simulink model "CryoDet6"  (R2015a)
settings: Solver=ode45  SolverMode=SingleTasking  StartTime=0.0  StopTime=1e-3  MaxStep=Tclk/8  RelTol=1e-3
values from neighbouring files (symbols this model uses):
  Fclk = Fadc/2    (= 185000000)    [setupCryoFPGA.m]    (also in setupCryoNew.m)
  noise = exp(1i*phi)    [setupCryoFPGA.m]    (also in setupCryoNew.m = exp(2i*pi*rand(1, noiseLen)))
  noiseLen = 128    [setupCryoFPGA.m]    (also in setupCryoNew.m)
  noiseSteps = 32    [setupCryoFPGA.m]    (also in setupCryoNew.m)
  notch = tf( [1 a*wNotch/Q wNotch^2], [1 wNotch/Q wNotch^2])    [setupCryoFPGA.m]    (also in setupCryoNew.m)
  notch2 = tf( [1 a*wNotch/Q wNotch^2], [1 wNotch/Q wNotch^2])    [setupCryoFPGA.m]    (also in setupCryoNew.m)
  setupVers = 5    [setupCryoFPGA.m]    (also in setupCryoNew.m = 21)
  Tclk = 1/Fclk    (= 5.40540540541e-09)    [setupCryoFPGA.m]    (also in setupCryoNew.m)
  wTs1 = w1*Ts1    (= 0.0271705310581)    [setupCryoFPGA.m]
undefined symbols (not defined in the file or in its folder): AXI4, Lite, xlipgetpartsetting
libraries: xbsIndex_r4 x516, simulink x1
(part 3 of 6)

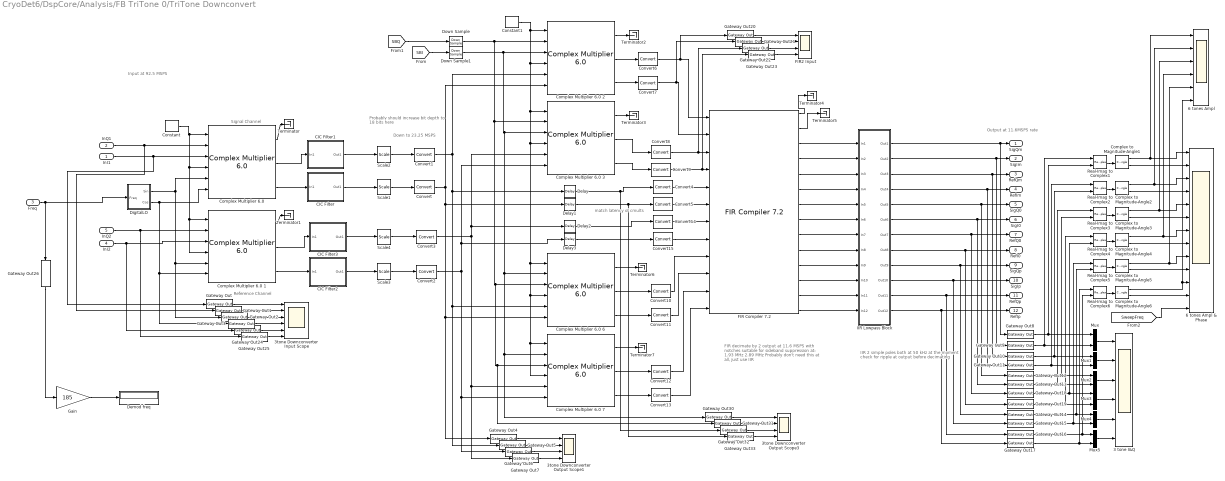
== system CryoDet6/DspCore/Analysis/FB TriTone 0/TriTone Downconvert ==
  note: Probably should increase bit depth
      | to 18 bits here
  note: IIR 2 simple poles
      | both at 50 kHz at the moment
      | check for ripple at output before decimating
  note: FIR decimate by 2
      | output at 11.6 MSPS
      | with notches suitable for
      | sideband suppression at:
      | 1.93 MHz
      | 2.89 MHz
      |
      | Probably don't need this at all, just use IIR
  note: Output at 11.6MSPS rate
  note: Down to 23.25 MSPS
  note: Input at 92.5 MSPS
  note: Reference Channel
  note: Signal Channel
  note: match latency
      | of cmults
  InI1 : Inport
  InQ1 : Inport  Port=2
  Freq : Inport  Port=3
  InI2 : Inport  Port=4
  InQ2 : Inport  Port=5
  3 tone I&Q : Scope  NumInputPorts=6
      settings: TimeRange=0.0002910432432432433  YMin=-0.008~-0.003~-0.15~-0.025~-0.0075~-0.0075  YMax=0.005~0.004~0.15~0.225~0.0075~0.01  SaveName=ScopeData7  MaxDataPoints=10000  SampleInput=on  SampleTime=Tclk
  3tone Downconverter Input Scope : Scope  NumInputPorts=6
      settings: TimeRange=1e-05  YMin=-0.75~-0.75~-1~-1~-0.5~-0.5  YMax=0.75~0.75~1~1~0.4~0.5  SaveName=ScopeData4
  3tone Downconverter Output Scope1 : Scope  NumInputPorts=4
      settings: TimeRange=0.000216172972972973  YMin=0.05~-0.2~-0.7000000000000001~-0.2  YMax=0.25~0.2~-0.2000000000000001~0.6000000000000001  SaveName=ScopeData6
  3tone Downconverter Output Scope3 : Scope  NumInputPorts=4
      settings: TimeRange=9.98918918918919e-06  YMin=-1~-1~-1~-1  YMax=1~1~1~1  SaveName=ScopeData13
  6 tones Ampl : Scope  NumInputPorts=6
      settings: TimeRange=0.0001119135135135135  YMin=0.00025~0.00026~0.182~0.279182~0.0002~0.00026  YMax=0.00175~0.00039~0.187~0.279184~0.0014~0.00039  SaveName=TonePandA1  DataFormat=Structure  MaxDataPoints=10000  SampleInput=on  SampleTime=Tclk*64
  6 tones Ampl & Phase : Scope  NumInputPorts=13
      settings: TimeRange=0.0001119135135135135  YMin=0.048259~0.825~0.0490775~-1.275~0.100188~0.5~0.502076~-3~0.05489~-0.5~0.0557525~-3.125~6.9966e+07  YMax=0.0482615~1~0.0490875~-1.125~0.100192~0.675~0.502082~-2.825~0.0549025~-0.325~0.0557625~-2.975~6.997e+07  SaveName=TonePandA  DataFormat=Structure  MaxDataPoints=10000  SampleInput=on  SampleTime=Tclk*16
  CIC Filter : Subsystem  mask(CIC Filter){input_bitwidth=20, input_binpt=16, filter_type=Decimator, rate_change=4, stages=3, m=1, pipeline=on}
      mask prompts: input_bitwidth "Input Bit Width"; input_binpt "Input Binary Point"; filter_type "Filter Type"; rate_change "Sample Rate Change"; stages "Number of Stages"; m "Differential Delay"; pipeline "Pipeline Differentiators"
      mask help: Cascaded Integrated Comb (CIC) Filter
      mask init:
      | % CIC Single Channel v1.0
      | % Set Block Logo
      | sav_gcb=gcb;
      | [bg,fg] = xlcmap('XBlock',0);
      | iPos = get_param(sav_gcb,'Position');
      | iWidth=iPos(3)-iPos(1); iHeight=iPos(4)-iPos(2);
      | iCx=iWidth/2;
      | iCy=iHeight/2;
      | [logoX, logoY] = xlogo(iPos);
      | 
      | % Determine previous filter type and number of stages
      | prev_stages_list = find_system(sav_gcb, 'lookUnderMasks', 'all', 'FollowLinks', 'on', 'Regexp', 'on', 'Name', '^Integrator*'); %this is a cell array
      | prev_stages = length(prev_stages_list);
      | 
      | prev_filter_list = find_system(sav_gcb, 'lookUnderMasks', 'all', 'FollowLinks', 'on', 'Regexp', 'on', 'Name', '^Up Sample*'); %this is a cell array
      | if (isempty(prev_filter_list))
      |     prev_filter_list = find_system(sav_gcb, 'lookUnderMasks', 'all', 'FollowLinks', 'on', 'Regexp', 'on', 'Name', '^Down Sample*'); %this is a cell array
      |     if (isempty(prev_filter_list))
      |         errordlg('Previous Filter Type could not be determined')
      |     else
      |         prev_filter_type = 2;
      |     end
      | else
      |     prev_filter_type = 1;
      | end
      |   
      |   
      | % Print label on the block
      | if(filter_type == 2)
      |    cic_str = sprintf('%d-Stage\n CIC\n%d:1 Decimator',stages, rate_change);
      | else
      |    cic_str = sprintf('%d-Stage\n CIC\n1:%d Interpolator',stages, rate_change);	
      | end
      | 
      | % Make sure the entered values for stages and channels are positive integers
      | nstages = round(sum(abs(stages)));
      | 
      | % issue an error if the number of stages entered is zero
      | if (nstages == 0)
      | 	nstages = prev_stages;
      | 	errordlg('Number of Stages must be more than zero')
      | end
      | 
      | if (nstages == prev_stages) & (filter_type == prev_filter_type)
      |     return
      | end
      | 
      | if(filter_type == 2) % Decimator
      |    if (prev_filter_type == 1) % was interpolator so turn to decimator
      |        for i= 2:prev_stages,
      | 	      delete_line(sav_gcb, ['Integrator' int2str(i-1) '/' int2str(1)], ['Integrator' int2str(i) '/' int2str(1)]);
      | 	      delete_line(sav_gcb, ['Differentiator' int2str(i-1) '/' int2str(1)], ['Differentiator' int2str(i) '/' int2str(1)]);
      |        end
      | 
      |        % disconnect the last blocks in the two sections
      |        delete_line(sav_gcb, ['Differentiator' int2str(prev_stages) '/' int2str(1)], ['Up Sample/1']);
      |        delete_line(sav_gcb, ['Integrator' int2str(prev_stages) '/' int2str(1)], 'Out1/1');
      | 	
      | 	   % delete the line from the Up sampler to the Integrator
      | 	   delete_line(sav_gcb, 'Up Sample/1', 'Integrator1/1'); 
      | 	   delete_line(sav_gcb, 'In1/1', 'Differentiator1/1'); 
      | 	   
      | 	   % Delete the Up Sampler and then replace with an Down Sampler
      | 	   pup = get_param([sav_gcb '/Up Sample'], 'position');
      | 	   delete_block([sav_gcb '/Up Sample']);
      | 	   load_system('xbsIndex_r4');
      | 	   add_block('xbsIndex_r4/Down Sample', [sav_gcb '/Down Sample'], 'sample_ratio', 'rate_change','sample_phase', 'First Value of Frame', 'position', [pup(1), pup(2), pup(3),pup(4)]);
      | 	   
      | 	   % Switch the Integrators and Decimators around
      | 	   for i=1:prev_stages,
      | 		   tempi = get_param([sav_gcb '/Integrator' int2str(i)], 'position');
      | 	       tempd = get_param([sav_gcb '/Differentiator' int2str(i)], 'position');
      | 		   set_param([sav_gcb '/Differentiator' int2str(i)], 'position', [tempi(1), tempi(2), tempi(3), tempi(4)], 'output_bitwidth', 'ceil(stages*log2(rate_change*m) + input_bitwidth)');
      | 		   set_param([sav_gcb '/Integrator' int2str(i)], 'position', [tempd(1), tempd(2), tempd(3), tempd(4)]);
      | 	   end
      | 	   	   	
      | 	   % add back in the lines
      |        add_line(sav_gcb, 'In1/1', 'Integrator1/1', 'autorouting', 'on');
      | 	   add_line(sav_gcb, ['Integrator' int2str(prev_stages) '/1'], 'Down Sample/1', 'autorouting', 'on');
      | 	   add_line(sav_gcb, 'Down Sample/1', 'Differentiator1/1', 'autorouting', 'on');
      | 	   add_line(sav_gcb, ['Differentiator' int2str(prev_stages) '/1'], 'Out1/1', 'autorouting', 'on');
      | 	   for i= 2:prev_stages,
      |           add_line(sav_gcb, ['Integrator' int2str(i-1) '/1'], ['Integrator' int2str(i) '/' int2str(1)], 'autorouting', 'on');
      |           add_line(sav_gcb, ['Differentiator' int2str(i-1) '/1'], ['Differentiator' int2str(i) '/' int2str(1)], 'autorouting', 'on');
      | 	   end
      | 		
      |        %Set the Output bit widths of Differentiator and Integrator stages
      |        set_param([sav_gcb '/Differentiator1'], 'output_bitwidth', 'ceil(stages*log2(rate_change*m) + input_bitwidth)');
      | 	   	   %Set the Output bit width of Integrator stages
      | 	   %Calculate the Interpolator Integrator Output Bit Growth
      |        for i= 1:prev_stages,
      | 			 j = nstages+i;
      | 	         set_param([sav_gcb '/Integrator' int2str(i)], 'output_bitwidth', 'ceil(stages*log2(rate_change*m) + input_bitwidth)');
      |              set_param([sav_gcb '/Differentiator' int2str(i)], 'output_bitwidth', 'ceil(stages*log2(rate_change*m) + input_bitwidth)');
      | 	   end
      | 	   
      |    end
      |    
      |    if (nstages ~= prev_stages)
      |     
      |        % disconnect all the wires from all the blocks
      |        for i= 2:prev_stages,
      | 	      delete_line(sav_gcb, ['Integrator' int2str(i-1) '/' int2str(1)], ['Integrator' int2str(i) '/' int2str(1)]);
      | 	      delete_line(sav_gcb, ['Differentiator' int2str(i-1) '/' int2str(1)], ['Differentiator' int2str(i) '/' int2str(1)]);
      |        end
      | 
      |        % disconnect the last blocks in the two sections
      |        delete_line(sav_gcb, ['Integrator' int2str(prev_stages) '/' int2str(1)], ['Down Sample/1']);
      |        delete_line(sav_gcb, ['Differentiator' int2str(prev_stages) '/' int2str(1)], 'Out1/1');
      | 	
      | 	   % delete the line from the down sampler to the differentiator
      | 	   delete_line(sav_gcb, 'Down Sample/1', 'Differentiator1/1');
      | 	
      | 	   % Remove all the blocks except the first one (as we always will have one)
      |        for i=2:prev_stages,
      | 		  delete_block([sav_gcb '/Differentiator' int2str(i)]);
      | 	      delete_block([sav_gcb '/Integrator' int2str(i)]);
      |        end
      | 	   
      | 	   %Set the Output bit width of Differentiator stages
      |        set_param([sav_gcb '/Differentiator1'], 'output_bitwidth', 'ceil(stages*log2(rate_change*m) + input_bitwidth)');
      | 	   
      | 	   % collect data on the position of existing blocks
      | 	   pi = get_param([sav_gcb '/Integrator1'], 'position');
      | 	   pd = get_param([sav_gcb '/Differentiator1'], 'position');
      | 	   set_param([sav_gcb '/Differentiator1'], 'position', [pi(1)+(nstages+1)*80, pd(2), pi(3)+(nstages+1)*80, pd(4)]);
      | 	   pd = get_param([sav_gcb '/Differentiator1'], 'position');
      | 	
      | 	   % move the current blocks to accomadate for new blocks to be added 
      | 	   pds = get_param([sav_gcb '/Down Sample'], 'position');
      | 	   set_param([sav_gcb '/Down Sample'], 'position', [pi(1)+(nstages)*80, pds(2), pi(3)+(nstages)*80, pds(4)]);
      | 	   
      | 	   po = get_param([sav_gcb '/Out1'], 'position');
      | 	   set_param([sav_gcb '/Out1'], 'position', [pd(1)+(nstages+1)*80, po(2), pd(1)+(po(3)-po(1))+(nstages+1)*80, po(4)]);	
      | 	
      | 	   % add back in the line between the Down Sampler and the 1st Differentiator
      |        add_line(sav_gcb, 'Down Sample/1', ['Differentiator1/' int2str(1)], 'autorouting', 'on');
      | 
      | 	   % Only add blocks if more than one stage is required
      | 	   if (nstages ~= 1)
      | 		
      | 	       % Add in a copy of the first block to make up the required number of stages
      |            for i=2:nstages,
      |                add_block([sav_gcb '/Integrator1'], [sav_gcb '/Integrator' int2str(i)], 'position', [pi(1)+(i-1)*80, pi(2), pi(3)+(i-1)*80, pi(4)]);
      | 		       add_block([sav_gcb '/Differentiator1'], [sav_gcb '/Differentiator' int2str(i)], 'position', [pd(1)+(i-1)*80, pd(2), pd(3)+(i-1)*80, pd(4)]);
      | 	       end
      | 		
      | 	       % Connect up the wires to each block use autorouting
      |            for i= 2:nstages,
      |  		       add_line(sav_gcb, ['Integrator' int2str(i-1) '/' int2str(1)], ['Integrator' int2str(i) '/' int2str(1)], 'autorouting', 'on');
      | 	           add_line(sav_gcb, ['Differentiator' int2str(i-1) '/' int2str(1)], ['Differentiator' int2str(i) '/' int2str(1)], 'autorouting', 'on');
      |            end
      | 	    end
      | 	       % Connect the last blocks in the two sections
      |            add_line(sav_gcb, ['Integrator' int2str(nstages) '/' int2str(1)], ['Down Sample/1'], 'autorouting', 'on');
      |            add_line(sav_gcb, ['Differentiator' int2str(nstages) '/' int2str(1)], ['Out1/1'], 'autorouting', 'on');
      |    end
      | 
      | else % Interpolator
      |    
      | 	
      | 	if (prev_filter_type == 2) % was decimator so turn to interpolator
      | 	
      | 	  % disconnect all the wires from all the blocks
      |        for i= 2:prev_stages,
      | 	      delete_line(sav_gcb, ['Integrator' int2str(i-1) '/' int2str(1)], ['Integrator' int2str(i) '/' int2str(1)]);
      | 	      delete_line(sav_gcb, ['Differentiator' int2str(i-1) '/' int2str(1)], ['Differentiator' int2str(i) '/' int2str(1)]);
      |        end
      | 
      |        % disconnect the last blocks in the two sections
      |        delete_line(sav_gcb, ['Integrator' int2str(prev_stages) '/' int2str(1)], ['Down Sample/1']);
      |        delete_line(sav_gcb, ['Differentiator' int2str(prev_stages) '/' int2str(1)], 'Out1/1');
      | 	
      | 	   % delete the line from the down sampler to the Differentiator
      | 	   delete_line(sav_gcb, 'Down Sample/1', 'Differentiator1/1'); 
      | 	   delete_line(sav_gcb, 'In1/1', 'Integrator1/1'); 
      | 	   
      | 	   % Delete the Down Sampler and then replace with a Up Sampler
      | 	   pdwn = get_param([sav_gcb '/Down Sample'], 'position');
      | 	   delete_block([sav_gcb '/Down Sample']);
      | 	   load_system('xbsIndex_r4');
      | 	   add_block('xbsIndex_r4/Up Sample', [sav_gcb '/Up Sample'], 'sample_ratio', 'rate_change', 'position', [pdwn(1), pdwn(2), pdwn(3), pdwn(4)]);
      | 	   
      | 	   % Switch the Integrators and Decimators around
      | 	   for i=1:prev_stages,
      | 		   tempi = get_param([sav_gcb '/Integrator' int2str(i)], 'position');
      | 	       tempd = get_param([sav_gcb '/Differentiator' int2str(i)], 'position');
      | 		   set_param([sav_gcb '/Differentiator' int2str(i)], 'position', [tempi(1), tempi(2), tempi(3), tempi(4)], 'output_bitwidth', [int2str(i) '+ input_bitwidth']);
      | 		   set_param([sav_gcb '/Integrator' int2str(i)], 'position', [tempd(1), tempd(2), tempd(3), tempd(4)]);
      | 	   end
      | 	   	   	
      | 	   % add back in the lines
      |        add_line(sav_gcb, 'In1/1', 'Differentiator1/1', 'autorouting', 'on');
      | 	   add_line(sav_gcb, ['Differentiator' int2str(prev_stages) '/1'], 'Up Sample/1', 'autorouting', 'on');
      | 	   add_line(sav_gcb, 'Up Sample/1', 'Integrator1/1', 'autorouting', 'on');
      | 	   add_line(sav_gcb, ['Integrator' int2str(prev_stages) '/1'], 'Out1/1', 'autorouting', 'on');
      | 	   for i= 2:prev_stages,
      |           add_line(sav_gcb, ['Integrator' int2str(i-1) '/1'], ['Integrator' int2str(i) '/1'], 'autorouting', 'on');
      |           add_line(sav_gcb, ['Differentiator' int2str(i-1) '/1'], ['Differentiator' int2str(i) '/1'], 'autorouting', 'on');
      | 	   end
      | 	   
      | 	   %Set the Output bit width of Integrator stages
      | 	   %Calculate the Interpolator Integrator Output Bit Growth
      |        for i= 1:prev_stages,
      | 			 j = nstages+i;
      | 	         set_param([sav_gcb '/Integrator' int2str(i)], 'output_bitwidth', ['ceil(log2(2^(2*stages-' int2str(j) ')*(rate_change*m)^(' int2str(j) '-stages)) + input_bitwidth)']);
      | 	   end
      | 		
      |    end
      |    
      | 	
      | 	if (nstages ~= prev_stages)
      |     
      |        % disconnect all the wires from all the blocks
      |        for i= 2:prev_stages,
      | 	      delete_line(sav_gcb, ['Integrator' int2str(i-1) '/' int2str(1)], ['Integrator' int2str(i) '/' int2str(1)]);
      | 	      delete_line(sav_gcb, ['Differentiator' int2str(i-1) '/' int2str(1)], ['Differentiator' int2str(i) '/' int2str(1)]);
      |        end
      | 
      |        % disconnect the last blocks in the two sections
      |        delete_line(sav_gcb, ['Differentiator' int2str(prev_stages) '/' int2str(1)], ['Up Sample/1']);
      |        delete_line(sav_gcb, ['Integrator' int2str(prev_stages) '/' int2str(1)], 'Out1/1');
      |        
      | 	
      | 	   % delete the line from the Up sampler to the Integrator1 for movement later
      | 	   delete_line(sav_gcb, 'Up Sample/1', 'Integrator1/1'); 
      | 	
      | 	   % Remove all the blocks except the first one (as we always will have one)
      |        for i=2:prev_stages,
      | 		  delete_block([sav_gcb '/Differentiator' int2str(i)]);
      | 	      delete_block([sav_gcb '/Integrator' int2str(i)]);
      |        end
      | 	
      | 	   %Set the Output bit width of first Differentiator stage (other are set as copies of this block)
      |        set_param([sav_gcb '/Differentiator1'], 'output_bitwidth', '1 + input_bitwidth');
      | 	   
      | 	   % collect data on the position of existing blocks
      | 	   pi = get_param([sav_gcb '/Integrator1'], 'position');
      | 	   pd = get_param([sav_gcb '/Differentiator1'], 'position');
      | 	   set_param([sav_gcb '/Integrator1'], 'position', [pd(1)+(nstages+1)*80, pi(2), pd(3)+(nstages+1)*80, pi(4)]);
      | 	   pi = get_param([sav_gcb '/Integrator1'], 'position');
      | 	
      | 	   % move the current blocks to accomadate for new blocks to be added 
      | 	   pus = get_param([sav_gcb '/Up Sample'], 'position');
      | 	   set_param([sav_gcb '/Up Sample'], 'position', [pd(1)+(nstages)*80, pus(2), pd(3)+(nstages)*80, pus(4)]);
      | 	
      | 	   po = get_param([sav_gcb '/Out1'], 'position');
      |        set_param([sav_gcb '/Out1'], 'position', [pi(1)+(nstages+1)*80, po(2), pi(1)+(po(3)-po(1))+(nstages+1)*80, po(4)]);	
      |       
      | 	
      | 	   % add back in the line between the Up Sampler and the 1st Integrator1
      | 	   add_line(sav_gcb, 'Up Sample/1', 'Integrator1/1', 'autorouting', 'on');
      | 	   
      | 	   % Only add blocks if more than one stage is required
      | 	   if (nstages ~= 1)
      | 		
      | 	       % Add in a copy of the first block to make up the required number of stages
      |            for i=2:nstages,
      |                add_block([sav_gcb '/Integrator1'], [sav_gcb '/Integrator' int2str(i)], 'position', [pi(1)+(i-1)*80, pi(2), pi(3)+(i-1)*80, pi(4)]);
      | 		       add_block([sav_gcb '/Differentiator1'], [sav_gcb '/Differentiator' int2str(i)], 'position', [pd(1)+(i-1)*80, pd(2), pd(3)+(i-1)*80, pd(4)], 'output_bitwidth', [int2str(i) '+ input_bitwidth']);
      | 	       end
      | 		
      | 	       % Connect up the wires to each block use autorouting
      |            for i= 2:nstages,
      |  		       add_line(sav_gcb, ['Integrator' int2str(i-1) '/' int2str(1)], ['Integrator' int2str(i) '/' int2str(1)], 'autorouting', 'on');
      | 	           add_line(sav_gcb, ['Differentiator' int2str(i-1) '/' int2str(1)], ['Differentiator' int2str(i) '/' int2str(1)], 'autorouting', 'on');
      |            end
      | 	    end
      | 	       % Connect the last blocks in the two sections
      |            add_line(sav_gcb, ['Differentiator' int2str(nstages) '/1'], ['Up Sample/1'], 'autorouting', 'on');
      |            add_line(sav_gcb, ['Integrator' int2str(nstages) '/1'], ['Out1/1'], 'autorouting', 'on');
      | 		   
      | 	     %Set the Output bit width of Integrator stages
      | 	     %Calculate the Interpolator Integrator Output Bit Growth
      |           for i= 1:nstages,
      | 			 j = nstages+i;
      | 	         set_param([sav_gcb '/Integrator' int2str(i)], 'output_bitwidth', ['ceil(log2(2^(2*stages-' int2str(j) ')*(rate_change*m)^(' int2str(j) '-stages)) + input_bitwidth)']);
      | 	      end
      |    end
      | 	  
      | end
      | 
      | 
      | % Set the pipelining to ON or OFF on the differentiators
      | if (pipeline == 0)
      | 	for i= 1:nstages
      | 		set_param([sav_gcb '/Differentiator' int2str(i), '/AddSub'], 'latency', '0')
      | 	end
      | else
      | 	for i= 1:nstages
      | 		set_param([sav_gcb '/Differentiator' int2str(i), '/AddSub'], 'latency' ,'1')
      | 	end
      | end
      settings: CopyFcn=set_param(gcb, 'MaskSelfModifiable', 'on', 'LinkStatus', 'none');
      mask Help: eval('');xlDoc('-book','sysgen','-topic','CIC_Filter');
      mask TypeOptions filter_type: Interpolator | Decimator
      mask TypeOptions m: 1 | 2 | 3 | 4
      mask Display:
      | patch([0 iWidth iWidth 0],[0 0 iHeight iHeight] , bg);
      | patch(logoX,logoY , fg);
      | plot([0 0 iWidth iWidth 0], [0 iHeight iHeight 0 0]);
      | disp(cic_str)
  CIC Filter1 : Subsystem  mask(CIC Filter){input_bitwidth=20, input_binpt=16, filter_type=Decimator, rate_change=4, stages=3, m=1, pipeline=on}
      mask prompts: input_bitwidth "Input Bit Width"; input_binpt "Input Binary Point"; filter_type "Filter Type"; rate_change "Sample Rate Change"; stages "Number of Stages"; m "Differential Delay"; pipeline "Pipeline Differentiators"
      mask help: Cascaded Integrated Comb (CIC) Filter
      mask init: same as CryoDet6/DspCore/Analysis/FB TriTone 0/TriTone Downconvert/CIC Filter
      settings: CopyFcn=set_param(gcb, 'MaskSelfModifiable', 'on', 'LinkStatus', 'none');
      mask Help: eval('');xlDoc('-book','sysgen','-topic','CIC_Filter');
      mask TypeOptions filter_type: Interpolator | Decimator
      mask TypeOptions m: 1 | 2 | 3 | 4
      mask Display:
      | patch([0 iWidth iWidth 0],[0 0 iHeight iHeight] , bg);
      | patch(logoX,logoY , fg);
      | plot([0 0 iWidth iWidth 0], [0 iHeight iHeight 0 0]);
      | disp(cic_str)
  CIC Filter2 : Subsystem  mask(CIC Filter){input_bitwidth=20, input_binpt=16, filter_type=Decimator, rate_change=4, stages=3, m=1, pipeline=on}
      mask prompts: input_bitwidth "Input Bit Width"; input_binpt "Input Binary Point"; filter_type "Filter Type"; rate_change "Sample Rate Change"; stages "Number of Stages"; m "Differential Delay"; pipeline "Pipeline Differentiators"
      mask help: Cascaded Integrated Comb (CIC) Filter
      mask init: same as CryoDet6/DspCore/Analysis/FB TriTone 0/TriTone Downconvert/CIC Filter
      settings: CopyFcn=set_param(gcb, 'MaskSelfModifiable', 'on', 'LinkStatus', 'none');
      mask Help: eval('');xlDoc('-book','sysgen','-topic','CIC_Filter');
      mask TypeOptions filter_type: Interpolator | Decimator
      mask TypeOptions m: 1 | 2 | 3 | 4
      mask Display:
      | patch([0 iWidth iWidth 0],[0 0 iHeight iHeight] , bg);
      | patch(logoX,logoY , fg);
      | plot([0 0 iWidth iWidth 0], [0 iHeight iHeight 0 0]);
      | disp(cic_str)
  CIC Filter3 : Subsystem  mask(CIC Filter){input_bitwidth=20, input_binpt=16, filter_type=Decimator, rate_change=4, stages=3, m=1, pipeline=on}
      mask prompts: input_bitwidth "Input Bit Width"; input_binpt "Input Binary Point"; filter_type "Filter Type"; rate_change "Sample Rate Change"; stages "Number of Stages"; m "Differential Delay"; pipeline "Pipeline Differentiators"
      mask help: Cascaded Integrated Comb (CIC) Filter
      mask init: same as CryoDet6/DspCore/Analysis/FB TriTone 0/TriTone Downconvert/CIC Filter
      settings: CopyFcn=set_param(gcb, 'MaskSelfModifiable', 'on', 'LinkStatus', 'none');
      mask Help: eval('');xlDoc('-book','sysgen','-topic','CIC_Filter');
      mask TypeOptions filter_type: Interpolator | Decimator
      mask TypeOptions m: 1 | 2 | 3 | 4
      mask Display:
      | patch([0 iWidth iWidth 0],[0 0 iHeight iHeight] , bg);
      | patch(logoX,logoY , fg);
      | plot([0 0 iWidth iWidth 0], [0 iHeight iHeight 0 0]);
      | disp(cic_str)
  "Complex Multiplier 6.0 " : xbsIndex_r4/Complex Multiplier 6.0   hasatlast=off  hasatuser=off  atuserwidth=1  hasbtlast=off  hasbtuser=off  btuserwidth=1  multtype=Use_Mults  optimizegoal=Resources  flowcontrol=NonBlocking  outputwidth=20  roundmode=Truncate  hasctrltlast=off  hasctrltuser=off  ctrltuserwidth=1  outtlastbehv=Null  latencyconfig=Automatic  minimumlatency=37  aclken=off  aresetn=off  trim_axipin_name=on  simulation_type=hybrid_sim  simulation_model=sysgen:cmpy_v6_0  data_path_portlist={ 's_axis_a_tdata_real', 's_axis_a_tdata_imag', 's_axis_b_tdata_real', 's_axis_b_tdata_imag', 's_axis_ctrl_tdata_rounding_bit', 'm_axis_dout_tdata_real', 'm_axis_dout_tdata_imag' }  aportwidth=63  bportwidth=63  ip_name=Complex Multiplier  ip_version=6.0  dsptool_ready=true  ipcore_usecache=true  ipcore_useipmodelcache=true  ipcore_verbose=false  ipcore_latency_parameter='minimumlatency'  wrapper_available=true  port_translation_map={ 'aclken' => 'en', 'aresetn' => 'rst'}  block_type=cmpy_v6_0
  Complex Multiplier 6.0 1 : xbsIndex_r4/Complex Multiplier 6.0   hasatlast=off  hasatuser=off  atuserwidth=1  hasbtlast=off  hasbtuser=off  btuserwidth=1  multtype=Use_Mults  optimizegoal=Resources  flowcontrol=NonBlocking  outputwidth=20  roundmode=Truncate  hasctrltlast=off  hasctrltuser=off  ctrltuserwidth=1  outtlastbehv=Null  latencyconfig=Automatic  minimumlatency=37  aclken=off  aresetn=off  trim_axipin_name=on  simulation_type=hybrid_sim  simulation_model=sysgen:cmpy_v6_0  data_path_portlist={ 's_axis_a_tdata_real', 's_axis_a_tdata_imag', 's_axis_b_tdata_real', 's_axis_b_tdata_imag', 's_axis_ctrl_tdata_rounding_bit', 'm_axis_dout_tdata_real', 'm_axis_dout_tdata_imag' }  aportwidth=63  bportwidth=63  ip_name=Complex Multiplier  ip_version=6.0  dsptool_ready=true  ipcore_usecache=true  ipcore_useipmodelcache=true  ipcore_verbose=false  ipcore_latency_parameter='minimumlatency'  wrapper_available=true  port_translation_map={ 'aclken' => 'en', 'aresetn' => 'rst'}  block_type=cmpy_v6_0
  Complex Multiplier 6.0 {2..3,6..7} (4 alike) : xbsIndex_r4/Complex Multiplier 6.0   hasatlast=off  hasatuser=off  atuserwidth=1  hasbtlast=off  hasbtuser=off  btuserwidth=1  multtype=Use_Mults  optimizegoal=Resources  flowcontrol=NonBlocking  outputwidth=19  roundmode=Truncate  hasctrltlast=off  hasctrltuser=off  ctrltuserwidth=1  outtlastbehv=Null  latencyconfig=Manual  minimumlatency=6  aclken=off  aresetn=off  trim_axipin_name=on  simulation_type=hybrid_sim  simulation_model=sysgen:cmpy_v6_0  data_path_portlist={ 's_axis_a_tdata_real', 's_axis_a_tdata_imag', 's_axis_b_tdata_real', 's_axis_b_tdata_imag', 's_axis_ctrl_tdata_rounding_bit', 'm_axis_dout_tdata_real', 'm_axis_dout_tdata_imag' }  aportwidth=63  bportwidth=63  ip_name=Complex Multiplier  ip_version=6.0  dsptool_ready=true  ipcore_usecache=true  ipcore_useipmodelcache=true  ipcore_verbose=false  ipcore_latency_parameter='minimumlatency'  wrapper_available=true  port_translation_map={ 'aclken' => 'en', 'aresetn' => 'rst'}  block_type=cmpy_v6_0
  Complex to Magnitude-Angle{1..6} (6 alike) : ComplexToMagnitudeAngle
  Constant : xbsIndex_r4/Constant  const=1  gui_display_data_type=Boolean  arith_type=Boolean  n_bits=16  bin_pt=14  preci_type=Single  exp_width=8  frac_width=24  explicit_period=off  period=1  equ=P=C  opselect=C  inp2=PCIN>>17  opr=+  inp1=P  carry=CIN  dbl_ovrd=off  block_type=constant
  Constant1 : xbsIndex_r4/Constant  const=1  gui_display_data_type=Boolean  arith_type=Boolean  n_bits=16  bin_pt=14  preci_type=Single  exp_width=8  frac_width=24  explicit_period=off  period=1  equ=P=C  opselect=C  inp2=PCIN>>17  opr=+  inp1=P  carry=CIN  dbl_ovrd=off  block_type=constant
  Convert{,1..3} (4 alike) : xbsIndex_r4/Convert  gui_display_data_type=Fixed-point  arith_type="Signed  (2's comp)"  n_bits=16  bin_pt=15  float_type=Single  exp_bits=8  fraction_bits=24  quantization=Truncate  overflow=Flag as error  en=off  latency=1  pipeline=off  dbl_ovrd=off  block_type=convert
  Convert{4..5,8..15} (10 alike) : xbsIndex_r4/Convert  gui_display_data_type=Fixed-point  arith_type="Signed  (2's comp)"  n_bits=16  bin_pt=14  float_type=Single  exp_bits=8  fraction_bits=24  quantization=Truncate  overflow=Wrap  en=off  latency=1  pipeline=off  dbl_ovrd=off  block_type=convert
  Convert6 : xbsIndex_r4/Convert  gui_display_data_type=Fixed-point  arith_type="Signed  (2's comp)"  n_bits=16  bin_pt=14  float_type=Single  exp_bits=8  fraction_bits=24  quantization=Truncate  overflow=Flag as error  en=off  latency=1  pipeline=off  dbl_ovrd=off  block_type=convert
  Convert7 : xbsIndex_r4/Convert  gui_display_data_type=Fixed-point  arith_type="Signed  (2's comp)"  n_bits=16  bin_pt=14  float_type=Single  exp_bits=8  fraction_bits=24  quantization=Truncate  overflow=Flag as error  en=off  latency=1  pipeline=off  dbl_ovrd=off  block_type=convert
  Delay{,1..3} (4 alike) : xbsIndex_r4/Delay  rst=off  infoeditControl=Selection of Reset will increase slice count due to use of real FFs and instead of SRLs  en=off  latency=6  reg_retiming=off  dbl_ovrd=off  block_type=delay
  Demod freq : Display
  DigitalLO : Subsystem
  Down Sample : xbsIndex_r4/Down Sample  sample_ratio=8  sample_phase=First Value of Frame  en=off  rst=off  latency=0  dbl_ovrd=off  block_type=dsamp
  Down Sample1 : xbsIndex_r4/Down Sample  sample_ratio=8  sample_phase=First Value of Frame  en=off  rst=off  latency=0  dbl_ovrd=off  block_type=dsamp
  "FIR Compiler 7.2 " : xbsIndex_r4/FIR Compiler 7.2   coefficientvector=FIR2  coefficient_sets=1  coefficient_reload=off  filter_type=Decimation  rate_change_type=Integer  interpolation_rate=1  decimation_rate=2  zero_pack_factor=1  channel_sequence=Basic  number_channels=1  pattern_list='P4-0,P4-1,P4-2,P4-3,P4-4'  number_paths=12  ratespecification=Maximum_Possible  sampleperiod=1  hardwareoversamplingrate=1  coefficient_sign=Unsigned  quantization=Quantize_Only  coefficient_width=16  bestprecision=on  coefficient_fractional_bits=19  coefficient_structure=Inferred  output_rounding_mode=Truncate_LSBs  output_width=18  filter_architecture=Systolic_Multiply_Accumulate  optimization_goal=Area  optimization_list='None'  data_buffer_type=Automatic  coefficient_buffer_type=Automatic  input_buffer_type=Automatic  output_buffer_type=Automatic  preference_for_other_storage=Automatic  multi_column_support=Automatic  columnconfig='7'  inter_column_pipe_length=4  data_has_tlast=Not_Required  m_data_has_tready=off  s_data_has_fifo=off  s_data_has_tuser=Not_Required  m_data_has_tuser=Not_Required  s_config_sync_mode=On_Vector  s_config_method=Single  num_reload_slots=1  has_aclken=off  has_aresetn=off  infoeditControl=ARESETn must be asserted for a minimum of 2 cycles  reset_data_vector=on  trim_axipin_name=on  simulation_type=hybrid_sim  simulation_model=sysgen:xfirv7_2_cmodel  data_path_portlist={ 's_axis_data_tdata', 'm_axis_data_tdata' }  passband_min=0.0  passband_max=0.5  stopband_min=0.5  stopband_max=1.0  filter_selection=1  gui_behaviour='Sysgen_GUI'  data_sign=Signed  data_width=16  data_fractional_bits=0  data_tuser_width=1  wrapper_available=true  ip_wrap_arbitrary_binary_point=true  ip_name=FIR Compiler  ip_version=7.2  dsptool_ready=true  ipcore_usecache=true  ipcore_useipmodelcache=true  port_translation_map={ 'aclken' => 'en', 'aresetn' => 'rst' }  run_core_at_system_period=true  ipcore_xco_need_fpga_part=true  block_type=fir_compiler_v7_2
      settings: infoedit=Maximum Possible : Maximizes oversampling rate. Abstracted input handshake (no s_data_tvalid) and automatic rate propagation.<br>Hardware Oversampling Rate : Specifies oversampling rate relative to the input sample period. Abstracted input handshake (no s_data_tvalid) and automatic rate propagation.<br>Input/Output Sample Period : Specifies absolute oversampling rate. No input handshake abstraction (exposes s_data_tvalid) and no rate propagation.
  FIR2 Input : Scope  NumInputPorts=4
      settings: TimeRange=2e-05  YMin=-2~-2~-1~-1  YMax=2~2~1~1  SaveName=ScopeData8
  Gain : Gain  Gain=185
  Gateway Out{,1..26,30..33} (31 alike) : xbsIndex_r4/Gateway Out  inherit_from_input=off  hdl_port=off  rows=1  columns=1  UseAsDAC=off  DACChannel='1'  interface=None  automatic_assignment=on  address_offset=hex2dec('00')  intf_name=''  intf_description=''  timing_constraint=None  locs_specified=off  LOCs={}  io_standard={}  block_type=gatewayout
  IIR Lowpass Block : Subsystem
  Mux{,1..5} (6 alike) : Mux  Inputs=2
  Real-Imag to Complex{1..6} (6 alike) : RealImagToComplex
  Scale{1..4} (4 alike) : xbsIndex_r4/Scale  scale_factor=-6  dbl_ovrd=off  block_type=scale
  Terminator{,1..7} (8 alike) : Terminator
  SigQm : Outport
  SigIm : Outport  Port=2
  RefQm : Outport  Port=3
  RefIm : Outport  Port=4
  SigQ0 : Outport  Port=5
  SigI0 : Outport  Port=6
  RefQ0 : Outport  Port=7
  RefI0 : Outport  Port=8
  SigQp : Outport  Port=9
  SigIp : Outport  Port=10
  RefQp : Outport  Port=11
  RefIp : Outport  Port=12
  wires:
  CIC Filter/1(Out1) -> Scale1/1
  CIC Filter1/1(Out1) -> Scale2/1
  CIC Filter2/1(Out1) -> Scale3/1
  CIC Filter3/1(Out1) -> Scale4/1
  Scale1/1 -> Convert/1
  Scale2/1 -> Convert1/1
  Scale4/1 -> Convert3/1
  InQ2/1 -> Gateway Out25/1, Complex Multiplier 6.0 1/2
  InQ1/1 -> Gateway Out1/1, "Complex Multiplier 6.0 "/2
  InI1/1 -> "Complex Multiplier 6.0 "/3, Gateway Out/1
  DigitalLO/1(Sin) -> Complex Multiplier 6.0 1/5, Gateway Out2/1, "Complex Multiplier 6.0 "/5
  InI2/1 -> Gateway Out24/1, Complex Multiplier 6.0 1/3
  Complex Multiplier 6.0 1/3 -> CIC Filter2/1(In1)
  "Complex Multiplier 6.0 "/3 -> CIC Filter/1(In1)
  "Complex Multiplier 6.0 "/2 -> CIC Filter1/1(In1)
  Constant/1 -> Complex Multiplier 6.0 1/4, Complex Multiplier 6.0 1/1, "Complex Multiplier 6.0 "/4, "Complex Multiplier 6.0 "/1
  Freq/1 -> DigitalLO/1(Freq), Gateway Out26/1
  Complex Multiplier 6.0 1/1 -> Terminator1/1
  "Complex Multiplier 6.0 "/1 -> Terminator/1
  Gateway Out/1 -> 3tone Downconverter Input Scope/1
  Gateway Out1/1 -> 3tone Downconverter Input Scope/2
  Gateway Out2/1 -> 3tone Downconverter Input Scope/3
  Gateway Out3/1 -> 3tone Downconverter Input Scope/4
  Gateway Out4/1 -> 3tone Downconverter Output Scope1/1
  Gateway Out5/1 -> 3tone Downconverter Output Scope1/2
  Gateway Out6/1 -> 3tone Downconverter Output Scope1/3
  Gateway Out7/1 -> 3tone Downconverter Output Scope1/4
  Complex Multiplier 6.0 2/1 -> Terminator2/1
  Complex Multiplier 6.0 3/1 -> Terminator3/1
  Complex Multiplier 6.0 6/1 -> Terminator6/1
  Complex Multiplier 6.0 7/1 -> Terminator7/1
  Constant1/1 -> Complex Multiplier 6.0 2/4, Complex Multiplier 6.0 6/1, Complex Multiplier 6.0 6/4, Complex Multiplier 6.0 7/1, Complex Multiplier 6.0 7/4, Complex Multiplier 6.0 3/4, Complex Multiplier 6.0 3/1, Complex Multiplier 6.0 2/1
  Complex Multiplier 6.0 2/3 -> Convert7/1
  "FIR Compiler 7.2 "/1 -> Terminator4/1
  "FIR Compiler 7.2 "/2 -> Terminator5/1
  Mux/1 -> 3 tone I&Q/1
  Mux1/1 -> 3 tone I&Q/2
  Mux2/1 -> 3 tone I&Q/3
  Gateway Out13/1 -> Real-Imag to Complex3/1, Mux2/2
  Gateway Out12/1 -> Real-Imag to Complex3/2, Mux2/1
  Gateway Out11/1 -> Real-Imag to Complex2/1, Mux1/2
  Gateway Out10/1 -> Real-Imag to Complex2/2, Mux1/1
  Gateway Out9/1 -> Real-Imag to Complex1/1, Mux/2
  Gateway Out8/1 -> Real-Imag to Complex1/2, Mux/1
  Scale3/1 -> Convert2/1
  Complex Multiplier 6.0 3/2 -> Convert8/1
  Complex Multiplier 6.0 3/3 -> Convert9/1
  Delay1/1 -> Gateway Out33/1, Convert5/1
  Delay2/1 -> Convert14/1
  Delay3/1 -> Convert15/1
  Complex Multiplier 6.0 6/2 -> Convert10/1
  Complex Multiplier 6.0 6/3 -> Convert11/1
  Complex Multiplier 6.0 7/2 -> Convert12/1
  Complex Multiplier 6.0 7/3 -> Convert13/1
  Mux3/1 -> 3 tone I&Q/4
  Mux4/1 -> 3 tone I&Q/5
  Mux5/1 -> 3 tone I&Q/6
  Gateway Out17/1 -> Real-Imag to Complex6/1, Mux5/2
  Gateway Out16/1 -> Real-Imag to Complex6/2, Mux5/1
  Gateway Out15/1 -> Real-Imag to Complex5/1, Mux4/2
  Gateway Out14/1 -> Real-Imag to Complex5/2, Mux4/1
  Gateway Out19/1 -> Real-Imag to Complex4/1, Mux3/2
  Gateway Out18/1 -> Real-Imag to Complex4/2, Mux3/1
  Convert/1 -> Complex Multiplier 6.0 2/6, Delay1/1, Complex Multiplier 6.0 6/6, Gateway Out4/1
  Convert3/1 -> Delay2/1, Complex Multiplier 6.0 3/5, Gateway Out7/1, Complex Multiplier 6.0 7/5
  Convert2/1 -> Gateway Out6/1, Complex Multiplier 6.0 7/6, Delay3/1, Complex Multiplier 6.0 3/6
  Delay/1 -> Gateway Out32/1, Convert4/1
  Complex Multiplier 6.0 2/2 -> Convert6/1
  Convert6/1 -> Gateway Out20/1, "FIR Compiler 7.2 "/1
  Convert7/1 -> Gateway Out21/1, "FIR Compiler 7.2 "/2
  Convert8/1 -> Gateway Out22/1, "FIR Compiler 7.2 "/3
  Convert9/1 -> Gateway Out23/1, "FIR Compiler 7.2 "/4
  Convert13/1 -> "FIR Compiler 7.2 "/12
  Convert12/1 -> "FIR Compiler 7.2 "/11
  Convert11/1 -> "FIR Compiler 7.2 "/10
  Convert10/1 -> "FIR Compiler 7.2 "/9
  Gateway Out20/1 -> FIR2 Input/1
  Gateway Out21/1 -> FIR2 Input/2
  Gateway Out22/1 -> FIR2 Input/3
  Gateway Out23/1 -> FIR2 Input/4
  [SBQ] -> Down Sample/1
  [SBI] -> Down Sample1/1
  Convert4/1 -> "FIR Compiler 7.2 "/5
  Convert15/1 -> "FIR Compiler 7.2 "/8
  Convert5/1 -> "FIR Compiler 7.2 "/6
  Convert14/1 -> "FIR Compiler 7.2 "/7
  Down Sample/1 -> Gateway Out31/1, Complex Multiplier 6.0 7/3, Complex Multiplier 6.0 6/3, Complex Multiplier 6.0 3/2, Complex Multiplier 6.0 2/2
  Down Sample1/1 -> Gateway Out30/1, Complex Multiplier 6.0 7/2, Complex Multiplier 6.0 6/2, Complex Multiplier 6.0 3/3, Complex Multiplier 6.0 2/3
  Gateway Out24/1 -> 3tone Downconverter Input Scope/5
  Gateway Out25/1 -> 3tone Downconverter Input Scope/6
  Complex Multiplier 6.0 1/2 -> CIC Filter3/1(In1)
  DigitalLO/2(Cos) -> Complex Multiplier 6.0 1/6, Gateway Out3/1, "Complex Multiplier 6.0 "/6
  Gateway Out30/1 -> 3tone Downconverter Output Scope3/1
  Gateway Out31/1 -> 3tone Downconverter Output Scope3/2
  Gateway Out32/1 -> 3tone Downconverter Output Scope3/3
  Gateway Out33/1 -> 3tone Downconverter Output Scope3/4
  Convert1/1 -> Delay/1, Complex Multiplier 6.0 6/5, Gateway Out5/1, Complex Multiplier 6.0 2/5
  IIR Lowpass Block/1(Out1) -> Gateway Out8/1, SigQm/1
  IIR Lowpass Block/12(Out12) -> Gateway Out17/1, RefIp/1
  IIR Lowpass Block/11(Out11) -> Gateway Out16/1, RefQp/1
  IIR Lowpass Block/10(Out10) -> Gateway Out15/1, SigIp/1
  IIR Lowpass Block/9(Out9) -> Gateway Out14/1, SigQp/1
  IIR Lowpass Block/8(Out8) -> Gateway Out19/1, RefI0/1
  IIR Lowpass Block/7(Out7) -> Gateway Out18/1, RefQ0/1
  IIR Lowpass Block/6(Out6) -> Gateway Out13/1, SigI0/1
  IIR Lowpass Block/5(Out5) -> Gateway Out12/1, SigQ0/1
  IIR Lowpass Block/4(Out4) -> Gateway Out11/1, RefIm/1
  IIR Lowpass Block/3(Out3) -> Gateway Out10/1, RefQm/1
  IIR Lowpass Block/2(Out2) -> Gateway Out9/1, SigIm/1
  "FIR Compiler 7.2 "/3 -> IIR Lowpass Block/1(In1)
  "FIR Compiler 7.2 "/4 -> IIR Lowpass Block/2(In2)
  "FIR Compiler 7.2 "/5 -> IIR Lowpass Block/3(In3)
  "FIR Compiler 7.2 "/6 -> IIR Lowpass Block/4(In4)
  "FIR Compiler 7.2 "/7 -> IIR Lowpass Block/5(In5)
  "FIR Compiler 7.2 "/8 -> IIR Lowpass Block/6(In6)
  "FIR Compiler 7.2 "/9 -> IIR Lowpass Block/7(In7)
  "FIR Compiler 7.2 "/10 -> IIR Lowpass Block/8(In8)
  "FIR Compiler 7.2 "/11 -> IIR Lowpass Block/9(In9)
  "FIR Compiler 7.2 "/12 -> IIR Lowpass Block/10(In10)
  "FIR Compiler 7.2 "/13 -> IIR Lowpass Block/11(In11)
  "FIR Compiler 7.2 "/14 -> IIR Lowpass Block/12(In12)
  Complex to Magnitude-Angle1/1 -> 6 tones Ampl/1, 6 tones Ampl & Phase/1
  Complex to Magnitude-Angle1/2 -> 6 tones Ampl & Phase/2
  Complex to Magnitude-Angle2/1 -> 6 tones Ampl/2, 6 tones Ampl & Phase/3
  Complex to Magnitude-Angle2/2 -> 6 tones Ampl & Phase/4
  Complex to Magnitude-Angle3/1 -> 6 tones Ampl/3, 6 tones Ampl & Phase/5
  Complex to Magnitude-Angle3/2 -> 6 tones Ampl & Phase/6
  Complex to Magnitude-Angle4/1 -> 6 tones Ampl/4, 6 tones Ampl & Phase/7
  Complex to Magnitude-Angle4/2 -> 6 tones Ampl & Phase/8
  Complex to Magnitude-Angle5/1 -> 6 tones Ampl/5, 6 tones Ampl & Phase/9
  Complex to Magnitude-Angle5/2 -> 6 tones Ampl & Phase/10
  Complex to Magnitude-Angle6/1 -> 6 tones Ampl/6, 6 tones Ampl & Phase/11
  Complex to Magnitude-Angle6/2 -> 6 tones Ampl & Phase/12
  Real-Imag to Complex1/1 -> Complex to Magnitude-Angle1/1
  Real-Imag to Complex2/1 -> Complex to Magnitude-Angle2/1
  Real-Imag to Complex3/1 -> Complex to Magnitude-Angle3/1
  Real-Imag to Complex4/1 -> Complex to Magnitude-Angle4/1
  Real-Imag to Complex5/1 -> Complex to Magnitude-Angle5/1
  Real-Imag to Complex6/1 -> Complex to Magnitude-Angle6/1
  [SweepFreq] -> 6 tones Ampl & Phase/13
  Gateway Out26/1 -> Gain/1
  Gain/1 -> Demod freq/1

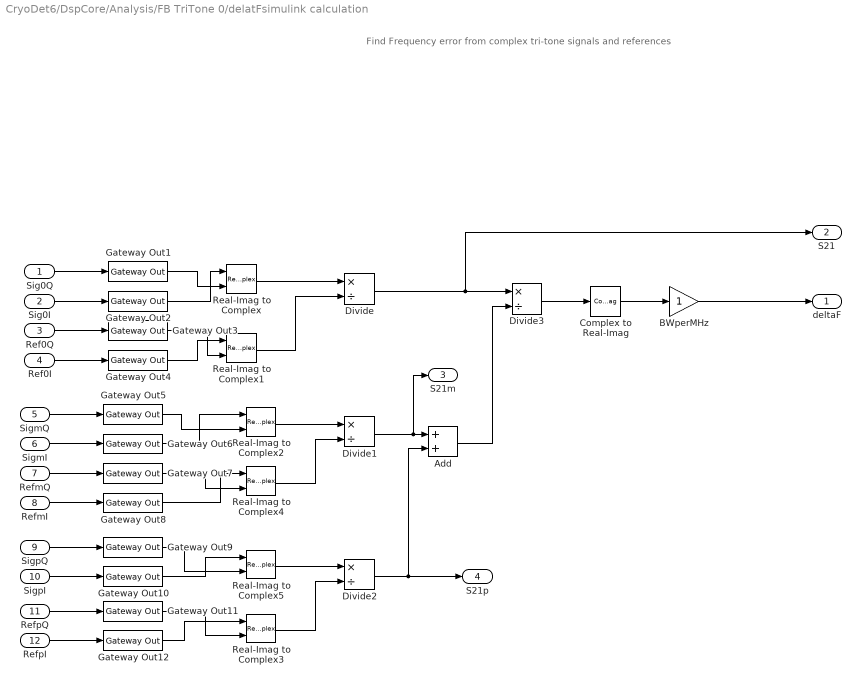
== system CryoDet6/DspCore/Analysis/FB TriTone 0/delatFsimulink calculation ==
  note: Find Frequency error from complex tri-tone signals and references
  Sig0Q : Inport
  Sig0I : Inport  Port=2
  Ref0Q : Inport  Port=3
  Ref0I : Inport  Port=4
  SigmQ : Inport  Port=5
  SigmI : Inport  Port=6
  RefmQ : Inport  Port=7
  RefmI : Inport  Port=8
  SigpQ : Inport  Port=9
  SigpI : Inport  Port=10
  RefpQ : Inport  Port=11
  RefpI : Inport  Port=12
  Add : Sum
  BWperMHz : Gain
  Complex to Real-Imag : ComplexToRealImag  Output=Imag
  Divide{,1..3} (4 alike) : Product  Inputs=*/
  Gateway Out{1..12} (12 alike) : xbsIndex_r4/Gateway Out  inherit_from_input=off  hdl_port=off  rows=1  columns=1  UseAsDAC=off  DACChannel='1'  interface=None  automatic_assignment=on  address_offset=hex2dec('00')  intf_name=''  intf_description=''  timing_constraint=None  locs_specified=off  LOCs={}  io_standard={}  block_type=gatewayout
  Real-Imag to Complex{,1..5} (6 alike) : RealImagToComplex
  deltaF : Outport
  S21 : Outport  Port=2
  S21m : Outport  Port=3
  S21p : Outport  Port=4
  wires:
  Sig0Q/1 -> Gateway Out1/1
  Sig0I/1 -> Gateway Out2/1
  Ref0Q/1 -> Gateway Out3/1
  Ref0I/1 -> Gateway Out4/1
  RefpI/1 -> Gateway Out12/1
  RefpQ/1 -> Gateway Out11/1
  SigpQ/1 -> Gateway Out9/1
  RefmI/1 -> Gateway Out8/1
  SigpI/1 -> Gateway Out10/1
  RefmQ/1 -> Gateway Out7/1
  SigmI/1 -> Gateway Out6/1
  SigmQ/1 -> Gateway Out5/1
  Gateway Out1/1 -> Real-Imag to Complex/2
  Gateway Out2/1 -> Real-Imag to Complex/1
  Gateway Out4/1 -> Real-Imag to Complex1/1
  Gateway Out3/1 -> Real-Imag to Complex1/2
  Real-Imag to Complex/1 -> Divide/1
  Real-Imag to Complex1/1 -> Divide/2
  Real-Imag to Complex2/1 -> Divide1/1
  Gateway Out6/1 -> Real-Imag to Complex2/1
  Gateway Out5/1 -> Real-Imag to Complex2/2
  Gateway Out11/1 -> Real-Imag to Complex3/2
  Gateway Out12/1 -> Real-Imag to Complex3/1
  Gateway Out7/1 -> Real-Imag to Complex4/2
  Gateway Out8/1 -> Real-Imag to Complex4/1
  Gateway Out10/1 -> Real-Imag to Complex5/1
  Gateway Out9/1 -> Real-Imag to Complex5/2
  Divide1/1 -> S21m/1, Add/1
  Divide2/1 -> S21p/1, Add/2
  Divide/1 -> S21/1, Divide3/1
  Add/1 -> Divide3/2
  Divide3/1 -> Complex to Real-Imag/1
  BWperMHz/1 -> deltaF/1
  Complex to Real-Imag/1 -> BWperMHz/1
  Real-Imag to Complex4/1 -> Divide1/2
  Real-Imag to Complex3/1 -> Divide2/2
  Real-Imag to Complex5/1 -> Divide2/1
